simulink model "TwoWheelModel"  (R2019b)
settings: Solver=FixedStepAuto  StartTime=0.0  StopTime=10.0  RelTol=1e-3
undefined symbols (not defined in the file): Rl, Rr, theta0, W, x0, y0
settings Model: Creator=r720r  LastModifiedBy=r720r

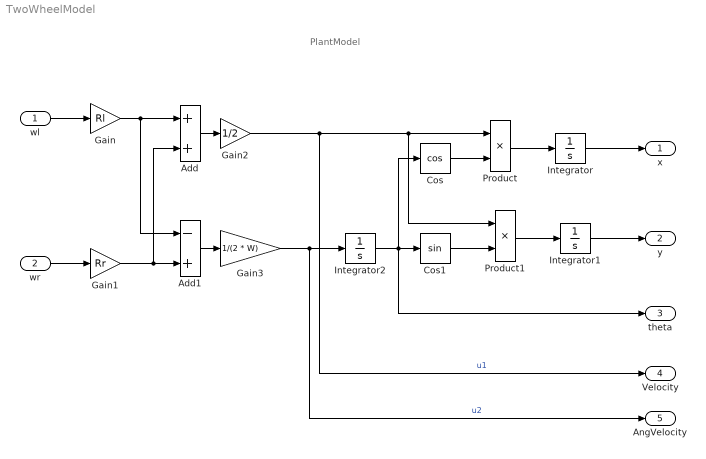
== system TwoWheelModel ==
  note: PlantModel
  wl : Inport
  wr : Inport  Port=2
  Add : Sum
  Add1 : Sum  Inputs=-+
  Cos : Trigonometry  Operator=cos
  Cos1 : Trigonometry
  Gain : Gain  Gain=Rl
  Gain1 : Gain  Gain=Rr
  Gain2 : Gain  Gain=1/2
  Gain3 : Gain  Gain=1/(2 * W)
  Integrator : Integrator  InitialCondition=x0
  Integrator1 : Integrator  InitialCondition=y0
  Integrator2 : Integrator  InitialCondition=theta0
  Product : Product
  Product1 : Product
  x : Outport
  y : Outport  Port=2
  theta : Outport  Port=3
  Velocity : Outport  Port=4
  AngVelocity : Outport  Port=5
  wires:
  Integrator/1 -> x/1
  wl/1 -> Gain/1
  Product/1 -> Integrator/1
  Gain/1 -> Add1/1, Add/1
  wr/1 -> Gain1/1
  Gain1/1 -> Add/2, Add1/2
  Add/1 -> Gain2/1
  Gain2/1 -> Velocity/1, Product1/1, Product/1  "u1"
  Add1/1 -> Gain3/1
  Gain3/1 -> Integrator2/1, AngVelocity/1  "u2"
  Integrator2/1 -> theta/1, Cos1/1, Cos/1
  Cos/1 -> Product/2
  Cos1/1 -> Product1/2
  Product1/1 -> Integrator1/1
  Integrator1/1 -> y/1
